simulink model "models1"  (R2020b)
settings: Solver=VariableStepAuto  StartTime=0.0  StopTime=10.0  RelTol=1e-3
settings Model: Creator=User  LastModifiedBy=User

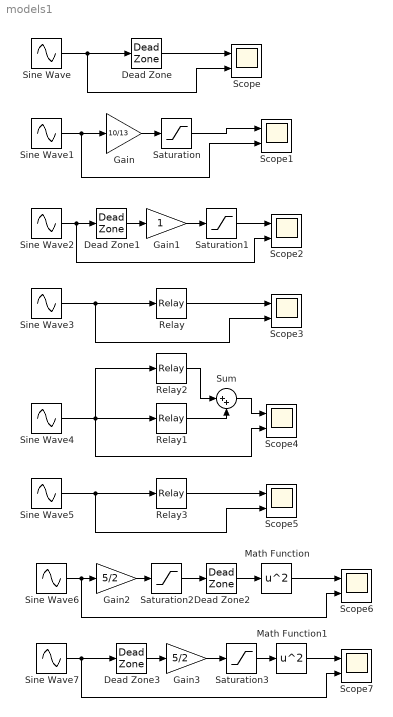
== system models1 ==
  Dead Zone : DeadZone  LowerValue=-0.1  UpperValue=0.1  SaturateOnIntegerOverflow=on
  Dead Zone1 : DeadZone  LowerValue=-0.1  UpperValue=0.1  SaturateOnIntegerOverflow=on
  Dead Zone2 : DeadZone  SaturateOnIntegerOverflow=on
  Dead Zone3 : DeadZone  SaturateOnIntegerOverflow=on
  Gain : Gain  Gain=10/13
  Gain1 : Gain
  Gain2 : Gain  Gain=5/2
  Gain3 : Gain  Gain=5/2
  Math Function : Math  Operator=square  SaturateOnIntegerOverflow=on
  Math Function1 : Math  Operator=square  SaturateOnIntegerOverflow=on
  Relay : Relay  OnSwitchValue=0  OffSwitchValue=0  OnOutputValue=0.4  OffOutputValue=-0.4
  Relay1 : Relay  OnSwitchValue=0.1  OffSwitchValue=0.1
  Relay2 : Relay  OnSwitchValue=-0.1  OffSwitchValue=-0.1  OnOutputValue=0  OffOutputValue=-1
  Relay3 : Relay  OnSwitchValue=0.1  OffSwitchValue=-0.1  OffOutputValue=-1
  Saturation : Saturate  UpperLimit=1  LowerLimit=-1
  Saturation1 : Saturate
  Saturation2 : Saturate  UpperLimit=5  LowerLimit=-5
  Saturation3 : Saturate  UpperLimit=5  LowerLimit=-5
  Scope{,1..7} (8 alike) : Scope  NumInputPorts=2
  Sine Wave{,1..2,4..5} (5 alike) : Sin  Amplitude=2  SampleTime=0
  Sine Wave3 : Sin  Amplitude=2  Frequency=0.5  SampleTime=0
  Sine Wave6 : Sin  Amplitude=3  Frequency=pi/2  SampleTime=0
  Sine Wave7 : Sin  Amplitude=3  Frequency=pi/2  SampleTime=0
  Sum : Sum  Inputs=|++
  wires:
  Sine Wave/1 -> Scope/2, Dead Zone/1
  Dead Zone/1 -> Scope/1
  Gain/1 -> Saturation/1
  Saturation/1 -> Scope1/1
  Sine Wave1/1 -> Gain/1, Scope1/2
  Gain1/1 -> Saturation1/1
  Saturation1/1 -> Scope2/1
  Dead Zone1/1 -> Gain1/1
  Sine Wave2/1 -> Dead Zone1/1, Scope2/2
  Relay/1 -> Scope3/1
  Sine Wave3/1 -> Relay/1, Scope3/2
  Sum/1 -> Scope4/1
  Relay2/1 -> Sum/1
  Relay1/1 -> Sum/2
  Sine Wave4/1 -> Relay2/1, Scope4/2, Relay1/1
  Relay3/1 -> Scope5/1
  Sine Wave5/1 -> Relay3/1, Scope5/2
  Gain2/1 -> Saturation2/1
  Math Function/1 -> Scope6/1
  Saturation2/1 -> Dead Zone2/1
  Dead Zone2/1 -> Math Function/1
  Sine Wave6/1 -> Scope6/2, Gain2/1
  Dead Zone3/1 -> Gain3/1
  Saturation3/1 -> Math Function1/1
  Gain3/1 -> Saturation3/1
  Math Function1/1 -> Scope7/1
  Sine Wave7/1 -> Scope7/2, Dead Zone3/1
